simulink model "EV_thermal_charger_2015a_20200311"  (R2015a)
settings: Solver=ode3  StartTime=0.0  StopTime=1800  FixedStep=sampling_time  RelTol=1e-3
PreLoadFcn:
  | run('init_setting.m')
PostLoadFcn:
  | set_param(gcs, 'SimulationCommand', 'update');
  | load('save_param/save_P_Charger', 'P_Charger');
  | load('save_param/save_T_User_set_temp_degC','T_User_set_temp_degC');
  | load('save_param/save_ENV_PNT_PTTH_Temp_add_degC','ENV_PNT_PTTH_Temp_add_degC');
  | load('save_param/save_ENV_PNT_CABIN_Temp_add_degC','ENV_PNT_CABIN_Temp_add_degC');
  | load('save_param/save_ENV_PNT_PHI_Sunlight_W','ENV_PNT_PHI_Sunlight_W');
  | load('save_param/save_ENV_PNT_Outside_Temp_ini_degC','ENV_PNT_Outside_Temp_ini_degC');
undefined symbols (not defined in the file or in its folder): BK_PNT_Pow_UL, BK_PNT_ReGene_vel_limit_DN_kmph, BK_PNT_ReGene_vel_limit_UP_kmph, BK_PNT_Tau_brake, Brk_LL, Brk_PGain, Brk_UL, BT_PNT_Hi_C_pol_hi_batt, BT_PNT_Hi_Capa_hi_batt_F, BT_PNT_Hi_ocv_SOC_hi_batt_OCV_V_table, BT_PNT_Hi_ocv_SOC_hi_batt_OCV_V_table_x_SOC, BT_PNT_Hi_R_hi_batt_cell, BT_PNT_Hi_R_pol_hi_batt, BT_PNT_Hi_SOC_MAX_hi_batt, BT_PNT_Hi_SOC_MIN_hi_batt, BT_PNT_Hi_SOC_START_hi_batt, BT_PNT_Lo_Capa_lo_batt_F, BT_PNT_Lo_ocv_SOC_lo_batt_OCV_V_table, BT_PNT_Lo_ocv_SOC_lo_batt_OCV_V_table_x_SOC, BT_PNT_Lo_R_lo_batt_ohm, BT_PNT_Lo_SOC_MAX_lo_batt, BT_PNT_Lo_SOC_MIN_lo_batt, BT_PNT_Lo_SOC_START_lo_batt, BTTH_CNT_P_BT_Heater_W, BTTH_CNT_P_BT_Heater_W_x_BTCells_degC, BTTH_CNT_Voltage_BTFan_V, BTTH_CNT_Voltage_BTFan_V_x_BTCells_degC, BTTH_PNT_BT_Heat_Resi_KpW, BTTH_PNT_BT_Heat_Resi_KpW_x_Wind_m3ps, BTTH_PNT_BT_Heater2BTCells_Heat_Resi_KpW, BTTH_PNT_BT_Heater_Heat_Capa_JpK, BTTH_PNT_BTBlock2BTAir_Heat_Resi_KpW, BTTH_PNT_BTBlock_Heat_Capa_JpK, BTTH_PNT_BTCells2BTBlock_Heat_Resi_KpW, BTTH_PNT_BTCells_Heat_Capa_JpK, BTTH_PNT_v_BTFan_Wind_vel_mps, BTTH_PNT_v_BTFan_Wind_vel_mps_x_V_BTFan, CATH_CNT_P_Aircon_W_LL, CATH_CNT_P_Aircon_W_UL, CATH_CNT_P_Gain_Aircon, CATH_CNT_P_Gain_PTC_Heater, CATH_CNT_P_Gain_SeatHT, CATH_CNT_P_PTC_Heater, CATH_CNT_P_PTC_Heater_W_LL, CATH_CNT_P_PTC_Heater_W_UL, CATH_CNT_P_PTC_Heater_x_T_Outside_temp_degC, CATH_CNT_P_SeatHT_W_LL, CATH_CNT_P_SeatHT_W_UL, CATH_CNT_PGain_Temp_blowout, CATH_CNT_T_Aircon_Indoor_degC, CATH_CNT_T_Aircon_Indoor_degC_x_T_blowout_degC, CATH_CNT_T_PTC_Heater_degC_UL, CATH_CNT_T_SeatHT_Temp_degC, CATH_CNT_T_SeatHT_Temp_degC_x_T_blowout_degC, CATH_CNT_V_HVAC_Fan, CATH_CNT_V_HVAC_Fan_x_T_blowout_degC, CATH_CNT_V_RDFan_V, CATH_CNT_V_RDFan_x_P_Aircon_W, CATH_PNT_Air_Convection_Heat_Resi_KpW, CATH_PNT_Air_Convection_Heat_Resi_x_mps ... (+141)
undefined symbols (not defined in the file): ACC_D_Gain, ACC_I_Gain, ACC_P_Gain
libraries: METI_Lib_vehicle_model x52, simulink x35
(part 4 of 6)

== system EV_thermal_charger_2015a_20200311/Vehicle/VCU_CNT/PDfSOC ==
  note: 放電電力マップ
  note: 充電電力マップ
  SOC_BT_Hi_PNT_per : Inport
  PSoFin_map : Lookup_n-D  NumberOfTableDimensions=1  BreakpointsForDimension1=VCU_CNT_PSoFin_soc  BeginIndexSearchUsingPreviousIndexResult=on  Table=VCU_CNT_PSoFin_battpw  ExtrapMethod=Clip  UseLastTableValue=on  InternalRulePriority=Speed  RndMeth=Simplest  InputSameDT=on
  PSoFout_map : Lookup_n-D  NumberOfTableDimensions=1  BreakpointsForDimension1=VCU_CNT_PSoFout_soc  BeginIndexSearchUsingPreviousIndexResult=on  Table=VCU_CNT_PSoFout_battpw  ExtrapMethod=Clip  UseLastTableValue=on  InternalRulePriority=Speed  RndMeth=Simplest  InputSameDT=on
  PSoFin : Outport
  PSoFout : Outport  Port=2
  wires:
  PSoFout_map/1 -> PSoFout/1
  PSoFin_map/1 -> PSoFin/1
  SOC_BT_Hi_PNT_per/1 -> PSoFout_map/1, PSoFin_map/1

== system EV_thermal_charger_2015a_20200311/Vehicle/VCU_CNT/ReGenerativeBrake_Calc ==
  note: 回生ブレーキ
      | 推進力[N]
  note: 回生ブレーキ
      | モータートルク[N]
  v_VL_PNT_mps_1 : Inport
  open_break_Driver_per : Inport  Port=2
  Constant : Constant  Value=0
  Constant2 : Constant  Value=1/TM_PNT_ratio_MG2_gear
  Constant4 : Constant  Value=tire_r
  Constant5 : Constant  Value=BK_PNT_Pow_UL
  Constant9 : Constant  Value=1/DF_PNT_DF_gear
  Gain : Gain  Gain=-1
  Product1 : Product  Inputs=6
  Product2 : Product
  ReBrake_Limit_Lowspeed : Subsystem
  Saturation Dynamic : simulink/Discontinuities/Saturation Dynamic  OutMin=[]  OutMax=[]  OutDataTypeStr=Inherit: Same as second input  OutDataType=fixdt(1, 16)  OutScaling=2^-10  DoSatur=off
  eta_DF1 : Constant  Value=TM_PNT_eta_MG2_gear
  eta_DF2 : Constant  Value=DF_PNT_eta_DF
  per2F2 : Gain  Gain=1/100
  trq_R_brake_tgt : Outport
  wires:
  Saturation Dynamic/1 -> Product1/1
  Constant/1 -> Saturation Dynamic/1
  Gain/1 -> Saturation Dynamic/2
  per2F2/1 -> Product2/1
  Constant5/1 -> Product2/2
  Product2/1 -> Gain/1
  open_break_Driver_per/1 -> per2F2/1
  Constant4/1 -> Product1/2
  Constant9/1 -> Product1/3
  eta_DF2/1 -> Product1/4
  Product1/1 -> trq_R_brake_tgt/1
  Constant2/1 -> Product1/5
  eta_DF1/1 -> Product1/6
  v_VL_PNT_mps_1/1 -> ReBrake_Limit_Lowspeed/1(Vehicle_Speed_mps)
  ReBrake_Limit_Lowspeed/1(F_Brake_limit_lowspeed) -> Saturation Dynamic/3

== system EV_thermal_charger_2015a_20200311/Vehicle/VCU_CNT/trq_MG2_GuardCalc ==
  note: 回生側のトルク制限
  note: 加速側のトルク制限
  w_MG_PNT_radps : Inport
  PSoFin : Inport  Port=2
  PSoFout : Inport  Port=3
  P_HVAC_PNT_W : Inport  Port=4
  P_DCDC_PNT_W : Inport  Port=5
  Abs : Abs
  Divide_0wari : METI_Lib_vehicle_model/Divide_0wari
  Divide_0wari1 : METI_Lib_vehicle_model/Divide_0wari
  MinMax : MinMax  Function=max  Inputs=2
  MinMax1 : MinMax  Inputs=2
  MinMax2 : MinMax  Inputs=2
  MinMax3 : MinMax  Function=max  Inputs=2
  Subtract1 : Sum  Inputs=+--
  Subtract2 : Sum  Inputs=+--
  力行側出力上限 : Constant  Value=MG_CNT_Pmax_MG_Gene_W
  力行側定トルク回転数上限 : Constant  Value=MG_CNT_MG_Const_trq_Gene_radps
  回生側出力上限 : Constant  Value=MG_CNT_Pmin_MG_ReGene_W
  回生側定トルク回転数上限 : Constant  Value=MG_CNT_MG_Const_trq_ReGene_radps
  trq_MG2_UpperGuard : Outport
  trq_MG2_LowerGuard : Outport  Port=2
  wires:
  MinMax2/1 -> Divide_0wari1/1  "使用可能電力"
  w_MG_PNT_radps/1 -> Abs/1
  Divide_0wari1/1 -> trq_MG2_UpperGuard/1  "トルク上限"
  MinMax/1 -> Divide_0wari1/2, Divide_0wari/2
  Abs/1 -> MinMax/1
  MinMax1/1 -> MinMax/2
  PSoFout/1 -> Subtract1/1  "バッテリ放電電力上限値"
  P_HVAC_PNT_W/1 -> Subtract2/2, Subtract1/2
  MinMax3/1 -> Divide_0wari/1
  Divide_0wari/1 -> trq_MG2_LowerGuard/1
  PSoFin/1 -> Subtract2/1
  力行側定トルク回転数上限/1 -> MinMax1/1
  回生側定トルク回転数上限/1 -> MinMax1/2
  Subtract1/1 -> MinMax2/1  "使用可能電力"
  Subtract2/1 -> MinMax3/2
  力行側出力上限/1 -> MinMax2/2
  回生側出力上限/1 -> MinMax3/1
  P_DCDC_PNT_W/1 -> Subtract2/3, Subtract1/3

== system EV_thermal_charger_2015a_20200311/Vehicle/VCU_CNT/trq_MG2_tgtCalc2 ==
  note: ～回生協調ブレーキ時～
      | アクセルオフによる回生ブレーキトルクと
      | ブレーキ操作による回生ブレーキトルクを合算し
      | モーター要求トルクとする
  note: ～回生協調ブレーキ時～
      | モーター要求トルクから
      | アクセルオフによる回生ブレーキトルクを減算し
      | 実際に出力できているブレーキ操作による回生ブレーキトルクを算出
      | それを車両駆動力としてブレーキECUへ送信する
  User_Power_req : Inport
  w_MG_PNT_radps : Inport  Port=2
  trq_motor_UserAcc_tgt : Inport  Port=3
  trq_MG2_UpperGuard : Inport  Port=4
  trq_MG2_LowerGuard : Inport  Port=5
  trq_R_brake_tgt : Inport  Port=6
  Add : Sum
  Add1 : Sum  Inputs=+-
  Constant1 : Constant  Value=TM_PNT_ratio_MG2_gear
  Constant2 : Constant  Value=DF_PNT_DF_gear
  Constant4 : Constant  Value=1/tire_r
  Product1 : Product  Inputs=6
  Saturation Dynamic2 : simulink/Discontinuities/Saturation Dynamic  OutMin=[]  OutMax=[]  OutDataTypeStr=Inherit: Same as second input  OutDataType=fixdt(1, 16)  OutScaling=2^-10  DoSatur=off
  Saturation Dynamic4 : simulink/Discontinuities/Saturation Dynamic  OutMin=[]  OutMax=[]  OutDataTypeStr=Inherit: Same as second input  OutDataType=fixdt(1, 16)  OutScaling=2^-10  DoSatur=off
  Switch4 : Switch  Criteria=u2 > Threshold
  eta_DF1 : Constant  Value=1/DF_PNT_eta_DF
  eta_DF2 : Constant  Value=1/TM_PNT_eta_MG2_gear
  回転数上限超過時トルク制限処理 : Subsystem
  tgt_Trq_VCU_CNT_MG_Nm : Outport
  F_VCU_CNT_re_break_N : Outport  Port=2
  wires:
  Saturation Dynamic4/1 -> Add1/1, tgt_Trq_VCU_CNT_MG_Nm/1
  trq_MG2_LowerGuard/1 -> Saturation Dynamic2/3, Saturation Dynamic4/3
  回転数上限超過時トルク制限処理/1(flag_overrev) -> Switch4/2
  Add/1 -> Saturation Dynamic4/2
  trq_motor_UserAcc_tgt/1 -> 回転数上限超過時トルク制限処理/1(trq_MG2_tgt), Switch4/1
  trq_MG2_UpperGuard/1 -> Saturation Dynamic2/1, Saturation Dynamic4/1
  w_MG_PNT_radps/1 -> 回転数上限超過時トルク制限処理/2(w_ROT_motor)
  User_Power_req/1 -> 回転数上限超過時トルク制限処理/3(User_Power_req)
  回転数上限超過時トルク制限処理/2(trq_MG2_guarded) -> Switch4/3
  Add1/1 -> Product1/1
  Constant4/1 -> Product1/2
  Constant2/1 -> Product1/3
  eta_DF1/1 -> Product1/4
  Product1/1 -> F_VCU_CNT_re_break_N/1
  Switch4/1 -> Add/2, Saturation Dynamic2/2
  trq_R_brake_tgt/1 -> Add/1
  Saturation Dynamic2/1 -> Add1/2
  Constant1/1 -> Product1/5
  eta_DF2/1 -> Product1/6

== system EV_thermal_charger_2015a_20200311/Vehicle/VCU_CNT/ユーザ要求駆力算出 ==
  note: 低速時に目標出力が0にならないよう
      | 5km/h以下では車速を5km/hとして
      | 目標出力を計算するための
      | 速度切替処理
  note: モーター軸の要求トルク
  open_accel_Driver_per : Inport
  open_break_Driver_per : Inport  Port=2
  v_VL_PNT_mps_1 : Inport  Port=3
  Compare To Constant : simulink/Logic and Bit Operations/Compare To Constant  relop=<  const=VCU_CNT_trq_req_v_vehicle_th  OutDataTypeStr=boolean
  Compare To Constant1 : simulink/Logic and Bit Operations/Compare To Constant  relop=>  const=VCU_CNT_trq_req_brak_th  OutDataTypeStr=boolean
  Constant : Constant  Value=5
  Constant1 : Constant  Value=DF_PNT_DF_gear
  Constant2 : Constant  Value=TM_PNT_ratio_MG2_gear
  Constant3 : Constant  Value=VCU_CNT_trq_req_Gain_ON
  Constant4 : Constant  Value=1/tire_r
  Constant5 : Constant  Value=VCU_CNT_trq_req_Gain_OFF
  Gain1 : Gain  Gain=mps2kmph
  Logical Operator : Logic  AllPortsSameDT=off  OutDataTypeStr=boolean
  Product : Product
  Product1 : Product  Inputs=6
  Product3 : Product
  Relational Operator : RelationalOperator  Operator=>  OutDataTypeStr=boolean
  Switch : Switch  Criteria=u2 > Threshold  Threshold=0.5
  Switch1 : Switch  Criteria=u2 > Threshold  Threshold=0.5
  Transfer Fcn : TransferFcn  Denominator=[VCU_CNT_trq_req_delaytime 1]
  eta_DF1 : Constant  Value=DF_PNT_eta_DF
  eta_DF2 : Constant  Value=TM_PNT_eta_MG2_gear
  kmph2mps1 : Gain  Gain=kmph2mps
  mps2kmph : Gain  Gain=mps2kmph
  要求駆動トルク推定 : Lookup_n-D  BreakpointsForDimension1=VCU_CNT_trq_require_v_kmph  BreakpointsForDimension2=VCU_CNT_trq_require_accper  BeginIndexSearchUsingPreviousIndexResult=on  Table=VCU_CNT_trq_require_Nm  ExtrapMethod=Clip  InternalRulePriority=Speed  RndMeth=Simplest  InputSameDT=on
  P_vehicle_tgt : Outport
  trq_motor_UserAcc_tgt : Outport  Port=2
  wires:
  Switch/1 -> Product3/1
  Product3/1 -> P_vehicle_tgt/1
  Constant/1 -> kmph2mps1/1, Relational Operator/2
  mps2kmph/1 -> Relational Operator/1
  Relational Operator/1 -> Switch/2
  kmph2mps1/1 -> Switch/3
  Constant4/1 -> Product1/1
  Constant1/1 -> Product1/2
  eta_DF1/1 -> Product1/3
  Product1/1 -> Product3/2
  要求駆動トルク推定/1 -> Product1/6, Product/1
  Constant5/1 -> Switch1/1
  v_VL_PNT_mps_1/1 -> mps2kmph/1, Gain1/1, Switch/1
  open_break_Driver_per/1 -> Compare To Constant1/1
  Compare To Constant/1 -> Logical Operator/1
  Compare To Constant1/1 -> Logical Operator/2
  Logical Operator/1 -> Switch1/2
  Constant3/1 -> Switch1/3
  Switch1/1 -> Transfer Fcn/1
  Transfer Fcn/1 -> Product/2
  Product/1 -> trq_motor_UserAcc_tgt/1
  Gain1/1 -> 要求駆動トルク推定/1, Compare To Constant/1
  open_accel_Driver_per/1 -> 要求駆動トルク推定/2
  Constant2/1 -> Product1/4
  eta_DF2/1 -> Product1/5

== system EV_thermal_charger_2015a_20200311/Vehicle/VL_PNT/cal_Hill_Climbing_Resi ==
  note: 登坂抵抗
  In1 : Inport
  Constant2 : Constant  Value=g
  Constant3 : Constant  Value=M
  Gain : Gain  Gain=deg2rad
  Product1 : Product
  Product3 : Product
  Trigonometric Function : Trigonometry
  Out1 : Outport
  wires:
  Trigonometric Function/1 -> Product1/2
  Product1/1 -> Out1/1
  Product3/1 -> Product1/1
  Gain/1 -> Trigonometric Function/1
  Constant2/1 -> Product3/2
  Constant3/1 -> Product3/1
  In1/1 -> Gain/1

== system EV_thermal_charger_2015a_20200311/Driver/Caliculate_Opeining_Accel/FB/Filter ==
  In1 : Inport
  Gain3 : Gain  Gain=10
  Gain4 : Gain  Gain=0.1
  Rounding Function : Rounding  Operator=round
  Out1 : Outport
  wires:
  Rounding Function/1 -> Gain4/1
  In1/1 -> Gain3/1
  Gain3/1 -> Rounding Function/1
  Gain4/1 -> Out1/1

== system EV_thermal_charger_2015a_20200311/Driver/Caliculate_Opeining_Accel/FF1/Subsystem ==
  Req_Force : Inport
  Upper_Acc_Force_Input : Inport  Port=2
  Upper_ACC_percent : Inport  Port=3
  Lower_Acc_Force_Input : Inport  Port=4
  Lower_Acc_percent : Inport  Port=5
  Add10 : Sum
  Add11 : Sum  Inputs=+-
  Add8 : Sum  Inputs=+-
  Add9 : Sum  Inputs=+-
  Compare To Zero1 : simulink/Logic and Bit Operations/Compare To Zero  relop=>  OutDataTypeStr=boolean
  Divide_0wari2 : METI_Lib_vehicle_model/Divide_0wari
  Product2 : Product
  Acc_percent_Out : Outport
  threshold_Out : Outport  Port=2
  wires:
  Compare To Zero1/1 -> threshold_Out/1
  Req_Force/1 -> Add9/1
  Lower_Acc_Force_Input/1 -> Add9/2, Add8/2
  Add11/1 -> Product2/2
  Lower_Acc_percent/1 -> Add10/2, Add11/2
  Upper_Acc_Force_Input/1 -> Add8/1
  Product2/1 -> Add10/1
  Add8/1 -> Divide_0wari2/2
  Divide_0wari2/1 -> Product2/1
  Add9/1 -> Compare To Zero1/1, Divide_0wari2/1
  Upper_ACC_percent/1 -> Add11/1
  Add10/1 -> Acc_percent_Out/1

== system EV_thermal_charger_2015a_20200311/Driver/Caliculate_Opeining_Accel/FF1/Subsystem1 ==
  Req_Force : Inport
  Upper_Acc_Force_Input : Inport  Port=2
  Upper_ACC_percent : Inport  Port=3
  Lower_Acc_Force_Input : Inport  Port=4
  Lower_Acc_percent : Inport  Port=5
  Add10 : Sum
  Add11 : Sum  Inputs=+-
  Add8 : Sum  Inputs=+-
  Add9 : Sum  Inputs=+-
  Compare To Zero1 : simulink/Logic and Bit Operations/Compare To Zero  relop=>  OutDataTypeStr=boolean
  Divide_0wari2 : METI_Lib_vehicle_model/Divide_0wari
  Product2 : Product
  Acc_percent_Out : Outport
  threshold_Out : Outport  Port=2
  wires:
  Compare To Zero1/1 -> threshold_Out/1
  Req_Force/1 -> Add9/1
  Lower_Acc_Force_Input/1 -> Add9/2, Add8/2
  Add11/1 -> Product2/2
  Lower_Acc_percent/1 -> Add10/2, Add11/2
  Upper_Acc_Force_Input/1 -> Add8/1
  Product2/1 -> Add10/1
  Add8/1 -> Divide_0wari2/2
  Divide_0wari2/1 -> Product2/1
  Add9/1 -> Compare To Zero1/1, Divide_0wari2/1
  Upper_ACC_percent/1 -> Add11/1
  Add10/1 -> Acc_percent_Out/1

== system EV_thermal_charger_2015a_20200311/Driver/Caliculate_Opeining_Accel/FF1/Subsystem2 ==
  Req_Force : Inport
  Upper_Acc_Force_Input : Inport  Port=2
  Upper_ACC_percent : Inport  Port=3
  Lower_Acc_Force_Input : Inport  Port=4
  Lower_Acc_percent : Inport  Port=5
  Add10 : Sum
  Add11 : Sum  Inputs=+-
  Add8 : Sum  Inputs=+-
  Add9 : Sum  Inputs=+-
  Compare To Zero1 : simulink/Logic and Bit Operations/Compare To Zero  relop=>  OutDataTypeStr=boolean
  Divide_0wari2 : METI_Lib_vehicle_model/Divide_0wari
  Product2 : Product
  Acc_percent_Out : Outport
  threshold_Out : Outport  Port=2
  wires:
  Compare To Zero1/1 -> threshold_Out/1
  Req_Force/1 -> Add9/1
  Lower_Acc_Force_Input/1 -> Add9/2, Add8/2
  Add11/1 -> Product2/2
  Lower_Acc_percent/1 -> Add10/2, Add11/2
  Upper_Acc_Force_Input/1 -> Add8/1
  Product2/1 -> Add10/1
  Add8/1 -> Divide_0wari2/2
  Divide_0wari2/1 -> Product2/1
  Add9/1 -> Compare To Zero1/1, Divide_0wari2/1
  Upper_ACC_percent/1 -> Add11/1
  Add10/1 -> Acc_percent_Out/1

== system EV_thermal_charger_2015a_20200311/Driver/Caliculate_Opeining_Accel/FF1/慣性 ==
  v_tgt : Inport
  Add : Sum
  Constant : Constant  Value=M
  Constant1 : Constant  Value=1/2
  Derivative : Derivative
  Derivative1 : Derivative
  Divide1 : Product  Inputs=***
  Memory : Memory
  F_Inertia : Outport
  wires:
  Divide1/1 -> F_Inertia/1
  v_tgt/1 -> Derivative/1, Memory/1
  Add/1 -> Divide1/2
  Derivative/1 -> Add/1
  Derivative1/1 -> Add/2
  Memory/1 -> Derivative1/1
  Constant1/1 -> Divide1/1
  Constant/1 -> Divide1/3

== system EV_thermal_charger_2015a_20200311/Driver/Caliculate_Opeining_Accel/FF1/空気抵抗 ==
  v_tgt : Inport
  V_wind : Constant  Value=0
  cal_Air_resi1 : METI_Lib_vehicle_model/vehicle_model/cal_Air_resi  Vel_max=200
  F_air_resi : Outport
  wires:
  cal_Air_resi1/1 -> F_air_resi/1
  V_wind/1 -> cal_Air_resi1/2
  v_tgt/1 -> cal_Air_resi1/1

== system EV_thermal_charger_2015a_20200311/Driver/Caliculate_Opeining_Accel/FF1/転がり抵抗 ==
  v_tgt : Inport
  cal_roll_resi : METI_Lib_vehicle_model/vehicle_model/cal_roll_resi  Myu_tire=myu  Vehicle_Mass=M  Gravi_acc=g
  F_rollresi : Outport
  wires:
  cal_roll_resi/1 -> F_rollresi/1
  v_tgt/1 -> cal_roll_resi/1

== system EV_thermal_charger_2015a_20200311/Vehicle/BTTH_PNT/BB_PNT/BTBlock_Heat_Capacity ==
  ini_T_Environment_Outside_degC : Inport
  PHI_BTBlock1_W : Inport  Port=2
  PHI_BTBlock2_W : Inport  Port=3
  Add : Sum
  Add1 : Sum
  Constant : Constant  Value=BTTH_PNT_BTBlock_Heat_Capa_JpK
  Divide : Product  Inputs=/*
  Integrator : Integrator
  degC->K : Subsystem
  T_BTBlock1_K : Outport
  T_BTBlock2_K : Outport  Port=2
  wires:
  PHI_BTBlock2_W/1 -> Add/2
  PHI_BTBlock1_W/1 -> Add/1
  Constant/1 -> Divide/1
  Add/1 -> Divide/2
  Divide/1 -> Integrator/1
  ini_T_Environment_Outside_degC/1 -> degC->K/1(degC)
  Integrator/1 -> Add1/2
  Add1/1 -> T_BTBlock1_K/1, T_BTBlock2_K/1
  degC->K/1(K) -> Add1/1

== system EV_thermal_charger_2015a_20200311/Vehicle/BTTH_PNT/BB_PNT/BT_Block2Air_Heat_Resistance ==
  T_ATM_PNT_BB_K : Inport
  T_BTBlock_Resi2_K : Inport  Port=2
  Add : Sum  Inputs=+-
  Constant : Constant  Value=BTTH_PNT_BTBlock2BTAir_Heat_Resi_KpW
  Divide : Product  Inputs=*/
  Gain : Gain  Gain=-1
  Gain1 : Gain
  PHI_BT2AIR_Resi1_W : Outport
  PHI_BTBlock_Resi2_W : Outport  Port=2
  wires:
  Constant/1 -> Divide/2
  Add/1 -> Divide/1
  Divide/1 -> Gain/1, Gain1/1
  Gain/1 -> PHI_BTBlock_Resi2_W/1
  T_BTBlock_Resi2_K/1 -> Add/1
  T_ATM_PNT_BB_K/1 -> Add/2
  Gain1/1 -> PHI_BT2AIR_Resi1_W/1

== system EV_thermal_charger_2015a_20200311/Vehicle/BTTH_PNT/BC_PNT/BTCells_Heat_Capacity ==
  ini_T_Environment_Outside_degC : Inport
  PHI_BTCells1_W : Inport  Port=2
  PHI_BTCells2_W : Inport  Port=3
  PHI_BTCells3_W : Inport  Port=4
  PHI_BTCells4_W : Inport  Port=5
  Add : Sum  Inputs=++++
  Add1 : Sum
  Constant : Constant  Value=BTTH_PNT_BTCells_Heat_Capa_JpK
  Divide : Product  Inputs=/*
  Integrator : Integrator
  degC->K : Subsystem
  T_BTCells1_K : Outport
  T_BTCells2_K : Outport  Port=2
  T_BTCells3_K : Outport  Port=3
  T_BTCells4_K : Outport  Port=4
  wires:
  PHI_BTCells1_W/1 -> Add/1
  Constant/1 -> Divide/1
  Add/1 -> Divide/2
  Divide/1 -> Integrator/1
  ini_T_Environment_Outside_degC/1 -> degC->K/1(degC)
  Integrator/1 -> Add1/2
  Add1/1 -> T_BTCells4_K/1, T_BTCells3_K/1, T_BTCells1_K/1, T_BTCells2_K/1
  degC->K/1(K) -> Add1/1
  PHI_BTCells2_W/1 -> Add/2
  PHI_BTCells3_W/1 -> Add/3
  PHI_BTCells4_W/1 -> Add/4

== system EV_thermal_charger_2015a_20200311/Vehicle/BTTH_PNT/BC_PNT/BT_Cells2BTBlock_Heat_Resistance ==
  T_BTBlock_Resi1_K : Inport
  T_BTCells_Resi2_K : Inport  Port=2
  Add : Sum  Inputs=+-
  Constant : Constant  Value=BTTH_PNT_BTCells2BTBlock_Heat_Resi_KpW
  Divide : Product  Inputs=*/
  Gain : Gain  Gain=-1
  Gain1 : Gain
  PHI_BTBlock_Resi1_W : Outport
  PHI_BTCells_Resi2_W : Outport  Port=2
  wires:
  Constant/1 -> Divide/2
  Add/1 -> Divide/1
  Divide/1 -> Gain/1, Gain1/1
  T_BTCells_Resi2_K/1 -> Add/1
  T_BTBlock_Resi1_K/1 -> Add/2
  Gain1/1 -> PHI_BTBlock_Resi1_W/1
  Gain/1 -> PHI_BTCells_Resi2_W/1

== system EV_thermal_charger_2015a_20200311/Vehicle/BTTH_PNT/BF_PNT/BTFan_Heat_Resistance ==
  "BTTH_PNT_BTFan_Heat_Resi_KpW " : Inport
  T_ATM_PNT_BF_K : Inport  Port=2
  T_BT_Fan_Resi2_K : Inport  Port=3
  Add : Sum  Inputs=+-
  Divide : Product  Inputs=*/
  Gain : Gain  Gain=-1
  Gain1 : Gain
  PHI_BT_Fan_Resi1_W : Outport
  PHI_BT_Fan_Resi2_W : Outport  Port=2
  wires:
  "BTTH_PNT_BTFan_Heat_Resi_KpW "/1 -> Divide/2
  Add/1 -> Divide/1
  Divide/1 -> Gain/1, Gain1/1
  Gain/1 -> PHI_BT_Fan_Resi2_W/1
  T_BT_Fan_Resi2_K/1 -> Add/1
  T_ATM_PNT_BF_K/1 -> Add/2
  Gain1/1 -> PHI_BT_Fan_Resi1_W/1

== system EV_thermal_charger_2015a_20200311/Vehicle/BTTH_PNT/BF_PNT/BT_Fan_Heat_Resi_Calc ==
  note: ラジエターファンの動作で
      | 発生する風速
  BTTH_PNT_Voltage_BTFan_V : Inport
  1-D Lookup Table : Lookup_n-D  NumberOfTableDimensions=1  BreakpointsForDimension1=BTTH_PNT_BT_Heat_Resi_KpW_x_Wind_m3ps  Table=BTTH_PNT_BT_Heat_Resi_KpW  InternalRulePriority=Speed  RndMeth=Simplest  InputSameDT=on
  1-D Lookup Table1 : Lookup_n-D  NumberOfTableDimensions=1  BreakpointsForDimension1=BTTH_PNT_v_BTFan_Wind_vel_mps_x_V_BTFan  Table=BTTH_PNT_v_BTFan_Wind_vel_mps  InternalRulePriority=Speed  RndMeth=Simplest  InputSameDT=on
  "BTTH_PNT_BTFan_Heat_Resi_KpW " : Outport
  wires:
  BTTH_PNT_Voltage_BTFan_V/1 -> 1-D Lookup Table1/1
  1-D Lookup Table/1 -> "BTTH_PNT_BTFan_Heat_Resi_KpW "/1
  1-D Lookup Table1/1 -> 1-D Lookup Table/1

== system EV_thermal_charger_2015a_20200311/Vehicle/BTTH_PNT/BH_PNT/BT_Heater ==
  T_BT_Heater_K : Inport
  tgt_P_BTTH_CNT_BTHeater_W : Inport  Port=2
  V_BT_Lo_PNT_V : Inport  Port=3
  Divide_0wari : METI_Lib_vehicle_model/Divide_0wari
  Gain : Gain  Gain=-1
  Terminator : Terminator
  PHI_BT_Heater_W : Outport
  I_BT_Heater_A : Outport  Port=2
  wires:
  Divide_0wari/1 -> Gain/1
  tgt_P_BTTH_CNT_BTHeater_W/1 -> PHI_BT_Heater_W/1, Divide_0wari/1
  V_BT_Lo_PNT_V/1 -> Divide_0wari/2
  T_BT_Heater_K/1 -> Terminator/1
  Gain/1 -> I_BT_Heater_A/1

== system EV_thermal_charger_2015a_20200311/Vehicle/BTTH_PNT/BH_PNT/BT_Heater2BTCells_Heat_Resistance ==
  T_BTCells_Resi1_K : Inport
  T_BT_Heater_Resi2_K : Inport  Port=2
  Add : Sum  Inputs=+-
  Constant : Constant  Value=BTTH_PNT_BT_Heater2BTCells_Heat_Resi_KpW
  Divide : Product  Inputs=*/
  Gain : Gain  Gain=-1
  Gain1 : Gain
  PHI_BTCells_Resi1_W : Outport
  PHI_BT_Heater_Resi2_W : Outport  Port=2
  wires:
  Constant/1 -> Divide/2
  Add/1 -> Divide/1
  Divide/1 -> Gain/1, Gain1/1
  Gain/1 -> PHI_BT_Heater_Resi2_W/1
  T_BT_Heater_Resi2_K/1 -> Add/1
  T_BTCells_Resi1_K/1 -> Add/2
  Gain1/1 -> PHI_BTCells_Resi1_W/1

== system EV_thermal_charger_2015a_20200311/Vehicle/BTTH_PNT/BH_PNT/BT_Heater_Heat_Capacity ==
  PHI_BTCells_Resi1_W : Inport
  PHI_BT_Heater1_W : Inport  Port=2
  PHI_BT_Heater2_W : Inport  Port=3
  Add : Sum
  Add1 : Sum
  Constant : Constant  Value=BTTH_PNT_BT_Heater_Heat_Capa_JpK
  Divide : Product  Inputs=/*
  Integrator : Integrator
  degC->K : Subsystem
  T_BT_Heater1_K : Outport
  T_BT_Heater2_K : Outport  Port=2
  wires:
  PHI_BT_Heater2_W/1 -> Add/2
  PHI_BT_Heater1_W/1 -> Add/1
  Constant/1 -> Divide/1
  Add/1 -> Divide/2
  Divide/1 -> Integrator/1
  PHI_BTCells_Resi1_W/1 -> degC->K/1(degC)
  Integrator/1 -> Add1/2
  Add1/1 -> T_BT_Heater2_K/1, T_BT_Heater1_K/1
  degC->K/1(K) -> Add1/1

== system EV_thermal_charger_2015a_20200311/Vehicle/BT_Hi_PNT/Cal_SOC/Subsystem4 ==
  In1 : Inport
  In2 : Inport  Port=2
  To Workspace : ToWorkspace  VariableName=SOC_LoBat  SampleTime=-1
      settings: Decimation=num_tws_mabiki
  To Workspace1 : ToWorkspace  VariableName=Asec_LoBat  SampleTime=-1
      settings: Decimation=num_tws_mabiki
  wires:
  In1/1 -> To Workspace/1
  In2/1 -> To Workspace1/1

== system EV_thermal_charger_2015a_20200311/Vehicle/CATH_CNT/Calc_Temp_Blowout/FB ==
  T_diff_temp_degC : Inport
  Constant : Constant  Value=CATH_CNT_PGain_Temp_blowout
  Product : Product
  Q_FB : Outport
  wires:
  T_diff_temp_degC/1 -> Product/1
  Product/1 -> Q_FB/1
  Constant/1 -> Product/2

== system EV_thermal_charger_2015a_20200311/Vehicle/CATH_CNT/Calc_Temp_Blowout/FF1 ==
  note: [m2K/W]
  note: ユルゲスの実験式による
      | 対流の熱伝達率[W/m2K]を逆数にして
      | 熱抵抗[m2K/W]にしたもの
  note: [m2K/W]
  note: ユルゲスの実験式による
      | 対流の熱伝達率[W/m2K]を逆数にして
      | 熱抵抗[m2K/W]にしたもの
  note: 室内の風速
  T_Outside_temp_degC : Inport
  T_CABIN_AIR_temp_degC : Inport  Port=2
  v_vehicle_mps : Inport  Port=3
  Abs : Abs
  Add : Sum
  Air_Convection_Heat_Resi : Lookup_n-D  NumberOfTableDimensions=1  BreakpointsForDimension1=CATH_PNT_Air_Convection_Heat_Resi_x_mps  Table=CATH_PNT_Air_Convection_Heat_Resi_KpW  InternalRulePriority=Speed  RndMeth=Simplest  InputSameDT=on
  Air_Convection_Heat_Resi1 : Lookup_n-D  NumberOfTableDimensions=1  BreakpointsForDimension1=CATH_PNT_Air_Convection_Heat_Resi_x_mps  Table=CATH_PNT_Air_Convection_Heat_Resi_KpW  InternalRulePriority=Speed  RndMeth=Simplest  InputSameDT=on
  Constant1 : Constant  Value=CATH_PNT_CABIN_Glass_S_m2
  Constant2 : Constant  Value=CATH_PNT_CABIN_Glass_S_m2
  Constant3 : Constant
  Divide : Product  Inputs=*/
  Divide1 : Product  Inputs=*/
  Divide2 : Product  Inputs=*/
  Subtract : Sum  Inputs=-+
  Q_Heat_Transfar : Outport
  wires:
  T_Outside_temp_degC/1 -> Subtract/1
  T_CABIN_AIR_temp_degC/1 -> Subtract/2
  Divide1/1 -> Q_Heat_Transfar/1
  Air_Convection_Heat_Resi/1 -> Divide/1
  Abs/1 -> Air_Convection_Heat_Resi/1
  Constant1/1 -> Divide/2
  v_vehicle_mps/1 -> Abs/1
  Subtract/1 -> Divide1/1
  Air_Convection_Heat_Resi1/1 -> Divide2/1
  Constant3/1 -> Air_Convection_Heat_Resi1/1
  Constant2/1 -> Divide2/2
  Divide/1 -> Add/1
  Divide2/1 -> Add/2
  Add/1 -> Divide1/2

== system EV_thermal_charger_2015a_20200311/Vehicle/CATH_PNT/CABIN/CABIN_AIR ==
  note: 車室空気の
      | 熱容量
  note: ヒートポンプからの
      | 熱量
  note: PTCヒータからの
      | 熱量
  note: シートヒータからの
      | 熱量
  note: 直射日光からの
      | 熱量
  note: ガラスを通した
      | 外気からの熱量
  note: 不透明壁からの
      | 赤外線輻射による熱量
  note: 不透明壁を通した
      | 外気からの熱量
  note: 乗員からの
      | 熱量
  Temp_ini1 : Inport
  PHI_CABIN_Aircon_W : Inport  Port=2
  PHI_CABIN_PTC_W : Inport  Port=3
  PHI_CABIN_SeatHT_W : Inport  Port=4
  PHI_CABIN_Human_W : Inport  Port=5
  PHI_CABIN_Sunlight_W : Inport  Port=6
  PHI_CABIN_Glass_W : Inport  Port=7
  PHI_CABIN_Wall_W : Inport  Port=8
  PHI_CABIN_Radiation_W : Inport  Port=9
  Add : Sum  Inputs=++++++++
  Add1 : Sum
  Constant : Constant  Value=CATH_PNT_CABIN_AIR_Heat_Capa_JpK
  Divide : Product  Inputs=/*
  Integrator : Integrator  LowerSaturationLimit=0
  degC->K : Subsystem
  T_CABIN_AIR_temp_K1 : Outport
  T_CABIN_Aicon_K : Outport  Port=2
  T_CABIN_PTC_K : Outport  Port=3
  T_CABIN_SeatHT_K : Outport  Port=4
  T_CABIN_Glass_K : Outport  Port=5
  T_CABIN_Sunlight_K : Outport  Port=6
  T_CABIN_Wall_K : Outport  Port=7
  T_CABIN_Radiation_K : Outport  Port=8
  T_CABIN_Human_K : Outport  Port=9
  wires:
  Add1/1 -> T_CABIN_Aicon_K/1, T_CABIN_PTC_K/1, T_CABIN_SeatHT_K/1, T_CABIN_Human_K/1, T_CABIN_Wall_K/1, T_CABIN_Radiation_K/1, T_CABIN_Glass_K/1, T_CABIN_Sunlight_K/1, T_CABIN_AIR_temp_K1/1
  Constant/1 -> Divide/1
  Add/1 -> Divide/2
  Divide/1 -> Integrator/1
  Temp_ini1/1 -> degC->K/1(degC)
  Integrator/1 -> Add1/2
  degC->K/1(K) -> Add1/1
  PHI_CABIN_Aircon_W/1 -> Add/1
  PHI_CABIN_PTC_W/1 -> Add/2
  PHI_CABIN_SeatHT_W/1 -> Add/3
  PHI_CABIN_Human_W/1 -> Add/4
  PHI_CABIN_Wall_W/1 -> Add/5
  PHI_CABIN_Radiation_W/1 -> Add/6
  PHI_CABIN_Glass_W/1 -> Add/7
  PHI_CABIN_Sunlight_W/1 -> Add/8

== system EV_thermal_charger_2015a_20200311/Vehicle/CATH_PNT/CABIN/GLASS ==
  note: 室内の風速
  V_vehicle_mps : Inport
  Temp_ini : Inport  Port=2
  T_GLASS2AIR_K : Inport  Port=3
  PHI_GLASS_Sunlight2_W : Inport  Port=4
  T_GLASS_CABIN_K : Inport  Port=5
  T_GLASS_Sunlight1_K : Inport  Port=6
  CABIN_Glass_Heat_Capacity : Subsystem
  CABIN_Glass_Heat_Resistance : Subsystem
  CABIN_Glass_Heat_Resistance1 : Subsystem
  Constant : Constant  Value=5
  PHI_GLASS2AIR_W : Outport
  T_GLASS_Sunlight2_K : Outport  Port=2
  PHI_GLASS_Sunlight1_W : Outport  Port=3
  PHI_GLASS_CABIN_W : Outport  Port=4
  wires:
  CABIN_Glass_Heat_Resistance/1(PHI_CABIN_Glass_Resi1_W) -> PHI_GLASS2AIR_W/1
  T_GLASS2AIR_K/1 -> CABIN_Glass_Heat_Resistance/2(T_CABIN_Glass_Resi1_K)
  CABIN_Glass_Heat_Capacity/2(T_CABIN_Glass1_K) -> CABIN_Glass_Heat_Resistance1/3(T_CABIN_Glass_Resi3_K)
  CABIN_Glass_Heat_Resistance1/2(PHI_CABIN_Glass_Resi3_W) -> CABIN_Glass_Heat_Capacity/2(PHI_CABIN_Glass1_W)
  CABIN_Glass_Heat_Capacity/1(T_CABIN_Glass2_K) -> CABIN_Glass_Heat_Resistance/3(T_CABIN_Glass_Resi2_K)
  CABIN_Glass_Heat_Resistance/2(PHI_CABIN_Glass_Resi2_W) -> CABIN_Glass_Heat_Capacity/3(PHI_CABIN_Glass2_W)
  PHI_GLASS_Sunlight2_W/1 -> PHI_GLASS_Sunlight1_W/1
  T_GLASS_Sunlight1_K/1 -> T_GLASS_Sunlight2_K/1
  Temp_ini/1 -> CABIN_Glass_Heat_Capacity/1(Temp_ini)
  T_GLASS_CABIN_K/1 -> CABIN_Glass_Heat_Resistance1/2(T_CABIN_Glass_Resi4_K)
  CABIN_Glass_Heat_Resistance1/1(PHI_CABIN_Glass_Resi4_W) -> PHI_GLASS_CABIN_W/1
  Constant/1 -> CABIN_Glass_Heat_Resistance1/1(V_wind)
  V_vehicle_mps/1 -> CABIN_Glass_Heat_Resistance/1(V_wind)

== system EV_thermal_charger_2015a_20200311/Vehicle/CATH_PNT/CABIN/Human_Thermal ==
  T_Human_Thermal_K : Inport
  Constant : Constant  Value=CATH_PNT_PHI_Human_body_W
  Terminator : Terminator
  PHI_Human_Thermal_W : Outport
  wires:
  Constant/1 -> PHI_Human_Thermal_W/1
  T_Human_Thermal_K/1 -> Terminator/1

== system EV_thermal_charger_2015a_20200311/Vehicle/CATH_PNT/CABIN/K->degC ==
  K : Inport
  Constant2 : Constant  Value=K2degC
  Sum : Sum  Inputs=++|
  degC : Outport
  wires:
  K/1 -> Sum/2
  Constant2/1 -> Sum/1
  Sum/1 -> degC/1

== system EV_thermal_charger_2015a_20200311/Vehicle/CATH_PNT/CABIN/K->degC1 ==
  K : Inport
  Constant2 : Constant  Value=K2degC
  Sum : Sum  Inputs=++|
  degC : Outport
  wires:
  K/1 -> Sum/2
  Constant2/1 -> Sum/1
  Sum/1 -> degC/1

== system EV_thermal_charger_2015a_20200311/Vehicle/CATH_PNT/CABIN/K->degC2 ==
  K : Inport
  Constant2 : Constant  Value=K2degC
  Sum : Sum  Inputs=++|
  degC : Outport
  wires:
  K/1 -> Sum/2
  Constant2/1 -> Sum/1
  Sum/1 -> degC/1

== system EV_thermal_charger_2015a_20200311/Vehicle/CATH_PNT/CABIN/K->degC3 ==
  K : Inport
  Constant2 : Constant  Value=K2degC
  Sum : Sum  Inputs=++|
  degC : Outport
  wires:
  K/1 -> Sum/2
  Constant2/1 -> Sum/1
  Sum/1 -> degC/1

== system EV_thermal_charger_2015a_20200311/Vehicle/CATH_PNT/CABIN/WALL ==
  note: 室内の風速
  V_vehicle_mps : Inport
  Temp_ini : Inport  Port=2
  T_WALL2AIR_K : Inport  Port=3
  PHI_WALL_Radiation_W : Inport  Port=4
  T_WALL_CABIN_K : Inport  Port=5
  T_WALL_Radiation1_K : Inport  Port=6
  CABIN_Wall_Heat_Capacity : Subsystem
  CABIN_Wall_Heat_Resistance : Subsystem
  CABIN_Wall_Heat_Resistance1 : Subsystem
  Constant1 : Constant  Value=5
  PHI_WALL2AIR_W : Outport
  T_WALL_Radiation_K : Outport  Port=2
  PHI_WALL_CABIN_W : Outport  Port=3
  PHI_WALL_Radiation1_W : Outport  Port=4
  wires:
  CABIN_Wall_Heat_Resistance/1(PHI_Wall_Resi1_W) -> PHI_WALL2AIR_W/1
  T_WALL2AIR_K/1 -> CABIN_Wall_Heat_Resistance/2(T_Wall_Resi1_K)
  CABIN_Wall_Heat_Capacity/2(T_CABIN_Wall1_K) -> CABIN_Wall_Heat_Resistance1/3(T_CABIN_Wall_Resi1_K)
  CABIN_Wall_Heat_Resistance1/2(PHI_CABIN_Wall_Resi1_W) -> CABIN_Wall_Heat_Capacity/2(PHI_CABIN_Wall1_W)
  CABIN_Wall_Heat_Capacity/1(T_CABIN_Wall2_K) -> CABIN_Wall_Heat_Resistance/3(T_Wall_Resi2_K)
  CABIN_Wall_Heat_Resistance/2(PHI_Wall_Resi2_W) -> CABIN_Wall_Heat_Capacity/3(PHI_CABIN_Wall2_W)
  Temp_ini/1 -> CABIN_Wall_Heat_Capacity/1(Temp_ini)
  T_WALL_CABIN_K/1 -> CABIN_Wall_Heat_Resistance1/2(T_CABIN_Wall_Resi2_K)
  CABIN_Wall_Heat_Resistance1/1(PHI_CABIN_Wall_Resi2_W) -> PHI_WALL_CABIN_W/1
  Constant1/1 -> CABIN_Wall_Heat_Resistance1/1(V_wind)
  V_vehicle_mps/1 -> CABIN_Wall_Heat_Resistance/1(V_wind)
  T_WALL_Radiation1_K/1 -> T_WALL_Radiation_K/1
  PHI_WALL_Radiation_W/1 -> PHI_WALL_Radiation1_W/1

== system EV_thermal_charger_2015a_20200311/Vehicle/CATH_PNT/HVAC/Aircon ==
  note: 室外機の
      | 熱容量
  note: 室内機の
      | 熱容量
  P_Heatpomp_Power : Inport
  Temp_ini : Inport  Port=2
  V_Aircon_V : Inport  Port=3
  PHI_Aircon_Outdoor1_W : Inport  Port=4
  PHI_Aircon_Indoor1_W : Inport  Port=5
  Aircon_Indoor_Unit_Heat_Capacity1 : Subsystem
  Aircon_Outdoor_Unit_Heat_Capacity : Subsystem
  Gain1 : Gain  Gain=-1
  K->degC : Subsystem
  K->degC1 : Subsystem
  Product1 : Product
  Switching_Air_Conditioning_Circuit : Subsystem
  T_Aircon_Outdoor_degC : Outport
  T_Aircon_Indoor_degC : Outport  Port=2
  T_Aircon_Outdoor1_K : Outport  Port=3
  T_Aircon_Indoor1_K : Outport  Port=4
  I_Aircon_A : Outport  Port=5
  tag scope: tScope_PHI_Aircon_Indoor1=global, tScope_PHI_Aircon_Outdoor1=global, tScope_P_Aircon=global
  wires:
  Aircon_Indoor_Unit_Heat_Capacity1/1(T_Aircon_Indoor2_K) -> T_Aircon_Indoor1_K/1, K->degC1/1(K)
  PHI_Aircon_Indoor1_W/1 -> [tScope_PHI_Aircon_Indoor1], Aircon_Indoor_Unit_Heat_Capacity1/3(PHI_Aircon_Indoor2_W)
  Aircon_Outdoor_Unit_Heat_Capacity/1(T_Aircon_Outdoor2_K) -> T_Aircon_Outdoor1_K/1, K->degC/1(K)
  PHI_Aircon_Outdoor1_W/1 -> Aircon_Outdoor_Unit_Heat_Capacity/3(PHI_Aircon_Outdoor2_W), [tScope_PHI_Aircon_Outdoor1]
  Temp_ini/1 -> Aircon_Outdoor_Unit_Heat_Capacity/1(Temp_ini), Aircon_Indoor_Unit_Heat_Capacity1/1(Temp_ini)
  K->degC/1(degC) -> T_Aircon_Outdoor_degC/1
  K->degC1/1(degC) -> T_Aircon_Indoor_degC/1
  Aircon_Outdoor_Unit_Heat_Capacity/2(T_Aircon_Outdoor3_K) -> Switching_Air_Conditioning_Circuit/4(T_Aircon_Outdoor4_K)
  Aircon_Indoor_Unit_Heat_Capacity1/2(T_Aircon_Indoor3_K) -> Switching_Air_Conditioning_Circuit/3(T_Aircon_Indoor4_K)
  P_Heatpomp_Power/1 -> Switching_Air_Conditioning_Circuit/2(P_Heatpomp_Power)
  V_Aircon_V/1 -> Switching_Air_Conditioning_Circuit/1(V_Compressor_V), Product1/1
  Switching_Air_Conditioning_Circuit/1(I_Compressor_A) -> I_Aircon_A/1, Gain1/1
  Product1/1 -> [tScope_P_Aircon]
  Gain1/1 -> Product1/2
  Switching_Air_Conditioning_Circuit/2(PHI_Aircon_Outdoor4_W) -> Aircon_Outdoor_Unit_Heat_Capacity/2(PHI_Aircon_Outdoor3_W)
  Switching_Air_Conditioning_Circuit/3(PHI_Aircon_Indoor4_W) -> Aircon_Indoor_Unit_Heat_Capacity1/2(PHI_Aircon_Indoor3_W)

== system EV_thermal_charger_2015a_20200311/Vehicle/CATH_PNT/HVAC/Aircon_Fan_Heat_Resi_Calc ==
  note: ラジエターファンの動作で
      | ラジエターコアに当たる風量
  CATH_PNT_Voltage_HVAC_Fan_V : Inport
  1-D Lookup Table : Lookup_n-D  NumberOfTableDimensions=1  BreakpointsForDimension1=CATH_PNT_HVAC_Heat_Resi_KpW_x_Wind_m3ps  Table=CATH_PNT_HVAC_Heat_Resi_KpW  InternalRulePriority=Speed  RndMeth=Simplest  InputSameDT=on
  1-D Lookup Table1 : Lookup_n-D  NumberOfTableDimensions=1  BreakpointsForDimension1=CATH_PNT_v_HVAC_Fan_Wind_vel_m3ps_x_V_HVAC_Fan  Table=CATH_PNT_v_HVAC_Fan_Wind_vel_m3ps  InternalRulePriority=Speed  RndMeth=Simplest  InputSameDT=on
  "HVAC_Fan_Heat_Resi_KpW " : Outport
  wires:
  CATH_PNT_Voltage_HVAC_Fan_V/1 -> 1-D Lookup Table1/1
  1-D Lookup Table/1 -> "HVAC_Fan_Heat_Resi_KpW "/1
  1-D Lookup Table1/1 -> 1-D Lookup Table/1

== system EV_thermal_charger_2015a_20200311/Vehicle/CATH_PNT/HVAC/Aircon_Heat_Resistance ==
  "Aircon_Heat_Resi_KpW " : Inport
  T_Aircon_Resi1_K : Inport  Port=2
  T_Aircon_Resi2_K : Inport  Port=3
  Add : Sum  Inputs=+-
  Divide : Product  Inputs=*/
  Gain : Gain  Gain=-1
  Gain1 : Gain
  PHI_Aircon_Resi1_W : Outport
  PHI_Aircon_Resi2_W : Outport  Port=2
  wires:
  "Aircon_Heat_Resi_KpW "/1 -> Divide/2
  Add/1 -> Divide/1
  Divide/1 -> Gain1/1, Gain/1
  Gain/1 -> PHI_Aircon_Resi2_W/1
  T_Aircon_Resi2_K/1 -> Add/1
  T_Aircon_Resi1_K/1 -> Add/2
  Gain1/1 -> PHI_Aircon_Resi1_W/1

== system EV_thermal_charger_2015a_20200311/Vehicle/CATH_PNT/HVAC/Aircon_Heat_Resistance1 ==
  "Aircon_Heat_Resi_KpW " : Inport
  T_Aircon_Resi3_K : Inport  Port=2
  T_Aircon_Resi4_K : Inport  Port=3
  Add : Sum  Inputs=+-
  Divide : Product  Inputs=*/
  Gain : Gain  Gain=-1
  Gain1 : Gain
  PHI_Aircon_Resi3_W : Outport
  PHI_Aircon_Resi4_W : Outport  Port=2
  wires:
  "Aircon_Heat_Resi_KpW "/1 -> Divide/2
  Add/1 -> Divide/1
  Divide/1 -> Gain1/1, Gain/1
  Gain/1 -> PHI_Aircon_Resi4_W/1
  T_Aircon_Resi4_K/1 -> Add/1
  T_Aircon_Resi3_K/1 -> Add/2
  Gain1/1 -> PHI_Aircon_Resi3_W/1

== system EV_thermal_charger_2015a_20200311/Vehicle/CATH_PNT/HVAC/PTC_Heater1 ==
  note: エアコン用PTCヒーター
      | 熱容量
  P_PTC_Heater_Power : Inport
  Temp_ini : Inport  Port=2
  V_PTC_Heater1_V : Inport  Port=3
  PHI_PTC_Heater1_W : Inport  Port=4
  K->degC : Subsystem
  PTC_Heater : Subsystem
  PTC_Heater_Heat_Capacity : Subsystem
  T_PTC_Heater_degC : Outport
  T_PTC_Heater1_K : Outport  Port=2
  I_PTC_Heater1_A : Outport  Port=3
  wires:
  PTC_Heater_Heat_Capacity/2(T_PTC_Heater3_K) -> PTC_Heater/3(T_PTC_Heater4_K)
  PTC_Heater_Heat_Capacity/1(T_PTC_Heater2_K) -> T_PTC_Heater1_K/1, K->degC/1(K)
  PHI_PTC_Heater1_W/1 -> PTC_Heater_Heat_Capacity/3(PHI_PTC_Heater2_W)
  Temp_ini/1 -> PTC_Heater_Heat_Capacity/1(Temp_ini)
  K->degC/1(degC) -> T_PTC_Heater_degC/1
  P_PTC_Heater_Power/1 -> PTC_Heater/1(P_PTC_Heater_Power)
  V_PTC_Heater1_V/1 -> PTC_Heater/2(V_PTC_Heater4_V)
  PTC_Heater/2(I_PTC_Heater4_A) -> I_PTC_Heater1_A/1
  PTC_Heater/1(PHI_PTC_Heater4_W) -> PTC_Heater_Heat_Capacity/2(PHI_PTC_Heater3_W)

== system EV_thermal_charger_2015a_20200311/Vehicle/CATH_PNT/HVAC/RDCoolant2Air_Heat_Resistance1 ==
  "Aircon_Air_Heat_Resi_KpW " : Inport
  T_Aircon_Air_Resi1_K : Inport  Port=2
  T_Aircon_Air_Resi2_K : Inport  Port=3
  Add : Sum  Inputs=+-
  Divide : Product  Inputs=*/
  Gain : Gain  Gain=-1
  Gain1 : Gain
  PHI_Aircon_Air_Resi1_W : Outport
  PHI_Aircon_Air_Resi2_W : Outport  Port=2
  wires:
  "Aircon_Air_Heat_Resi_KpW "/1 -> Divide/2
  Add/1 -> Divide/1
  Divide/1 -> Gain1/1, Gain/1
  Gain/1 -> PHI_Aircon_Air_Resi2_W/1
  T_Aircon_Air_Resi2_K/1 -> Add/1
  T_Aircon_Air_Resi1_K/1 -> Add/2
  Gain1/1 -> PHI_Aircon_Air_Resi1_W/1

== system EV_thermal_charger_2015a_20200311/Vehicle/CATH_PNT/Seat_Heater/K->degC ==
  K : Inport
  Constant2 : Constant  Value=K2degC
  Sum : Sum  Inputs=++|
  degC : Outport
  wires:
  K/1 -> Sum/2
  Constant2/1 -> Sum/1
  Sum/1 -> degC/1

== system EV_thermal_charger_2015a_20200311/Vehicle/CATH_PNT/Seat_Heater/SeatHT_Heat_Capacity ==
  Temp_ini : Inport
  PHI_SeatHT1_W : Inport  Port=2
  PHI_SeatHT2_W : Inport  Port=3
  Add : Sum
  Add1 : Sum
  Constant : Constant  Value=CATH_PNT_Seat_Heater_Capa_JpK
  Divide : Product  Inputs=/*
  Integrator : Integrator
  degC->K : Subsystem
  T_SeatHT2_K : Outport
  T_SeatHT1_K : Outport  Port=2
  wires:
  PHI_SeatHT2_W/1 -> Add/2
  PHI_SeatHT1_W/1 -> Add/1
  Constant/1 -> Divide/1
  Add/1 -> Divide/2
  Divide/1 -> Integrator/1
  Temp_ini/1 -> degC->K/1(degC)
  Integrator/1 -> Add1/2
  Add1/1 -> T_SeatHT1_K/1, T_SeatHT2_K/1
  degC->K/1(K) -> Add1/1

== system EV_thermal_charger_2015a_20200311/Vehicle/CATH_PNT/Seat_Heater/Seat_HT ==
  P_Seat_Heater_Power : Inport
  V_Seat_HT_V : Inport  Port=2
  T_Seat_HT_K : Inport  Port=3
  Divide_0wari : METI_Lib_vehicle_model/Divide_0wari
  Gain : Gain  Gain=-1
  Terminator : Terminator
  PHI_Seat_HT_W : Outport
  I_Seat_HT_A : Outport  Port=2
  wires:
  P_Seat_Heater_Power/1 -> PHI_Seat_HT_W/1, Divide_0wari/1
  V_Seat_HT_V/1 -> Divide_0wari/2
  Divide_0wari/1 -> Gain/1
  Gain/1 -> I_Seat_HT_A/1
  T_Seat_HT_K/1 -> Terminator/1

== system EV_thermal_charger_2015a_20200311/Vehicle/CATH_PNT/Seat_Heater/Seat_Heater_Heat_Resistance ==
  T_SeatHT_Resi2_K : Inport
  T_SeatHT_Resi1_K : Inport  Port=2
  Add : Sum  Inputs=+-
  Constant : Constant  Value=CATH_PNT_CABIN_SeatHT_Heat_Resi_KpW
  Divide : Product  Inputs=*/
  Gain : Gain  Gain=-1
  Gain1 : Gain
  PHI_SeatHT_Resi1_W : Outport
  PHI_SeatHT_Resi2_W : Outport  Port=2
  wires:
  Constant/1 -> Divide/2
  Add/1 -> Divide/1
  Divide/1 -> Gain1/1, Gain/1
  Gain/1 -> PHI_SeatHT_Resi2_W/1
  T_SeatHT_Resi2_K/1 -> Add/1
  T_SeatHT_Resi1_K/1 -> Add/2
  Gain1/1 -> PHI_SeatHT_Resi1_W/1

== system EV_thermal_charger_2015a_20200311/Vehicle/CHG_CNT/Charge_Current_calc/Initial_Charge ==
  In1 : Inport
  Action Port : ActionPort  ActionType=elseif
  Out1 : Outport
  wires:
  In1/1 -> Out1/1

== system EV_thermal_charger_2015a_20200311/Vehicle/CHG_CNT/Charge_Current_calc/Negotiation_time ==
  Action Port : ActionPort  ActionType=then
  Constant : Constant  Value=0
  Out1 : Outport
  wires:
  Constant/1 -> Out1/1

== system EV_thermal_charger_2015a_20200311/Vehicle/CHG_CNT/Charge_Current_calc/Normal_Charge ==
  note: 一定電流充電モード（CC)
      | 一定電力充電モード（CP)
      | 一定電圧充電モード（CV)
      | の三者で目標電流値を算出し、
      | その中で最も小さい電流値だったものを採用する。
  Maximum_Charge_Current_A : Inport
  Maximum_Charge_Power_W : Inport  Port=2
  Maximum_Charge_Voltage_V : Inport  Port=3
  Battery_Voltage_V : Inport  Port=4
  SOC_HiBatt : Inport  Port=5
  Maximum_Hi_Batt_SOC : Inport  Port=6
  Action Port : ActionPort  ActionType=else
  Constant_Current_Charge : Subsystem
  Constant_Power_Charge : Subsystem
  Constant_Voltage_Charge : Subsystem
  Memory : Memory
  MinMax : MinMax  Inputs=3
  Relational Operator : RelationalOperator  Operator===  OutDataTypeStr=boolean
  Current_tgt : Outport
  wires:
  Maximum_Charge_Current_A/1 -> Constant_Current_Charge/1(Maximum_Charge_Current_A), Constant_Voltage_Charge/1(Maximum_Charge_Current_A)
  MinMax/1 -> Relational Operator/1, Current_tgt/1
  Maximum_Charge_Power_W/1 -> Constant_Power_Charge/1(Maximum_Charge_Power_W)
  Constant_Current_Charge/1(Current_tgt) -> MinMax/1
  Battery_Voltage_V/1 -> Constant_Power_Charge/2(Battery_Voltage_V), Constant_Voltage_Charge/4(Battery_Voltage_V)
  Constant_Power_Charge/1(Current_tgt) -> MinMax/2
  Constant_Voltage_Charge/1(Current_tgt) -> Relational Operator/2, MinMax/3
  Memory/1 -> Constant_Voltage_Charge/5(old_mode)
  Relational Operator/1 -> Memory/1
  Maximum_Hi_Batt_SOC/1 -> Constant_Voltage_Charge/3(Maximum_Hi_Batt_SOC)
  Maximum_Charge_Voltage_V/1 -> Constant_Voltage_Charge/2(Maximum_Charge_Voltage_V)
  SOC_HiBatt/1 -> Constant_Current_Charge/2(SOC_HiBatt)

== system EV_thermal_charger_2015a_20200311/Vehicle/ELTH_PNT/INVTH_PNT/INVBlock2Air_Heat_Resistance ==
  T_INV2Air_Resi1_K : Inport
  T_INVBlock_Resi3_K : Inport  Port=2
  Add : Sum  Inputs=+-
  Constant : Constant  Value=ELTH_PNT_INVBlock2DFAir_Heat_Resi_KpW
  Divide : Product  Inputs=*/
  Gain : Gain  Gain=-1
  Gain1 : Gain
  PHI_INV2Air_Resi1_W : Outport
  PHI_INVBlock_Resi3_W : Outport  Port=2
  wires:
  Constant/1 -> Divide/2
  Add/1 -> Divide/1
  Divide/1 -> Gain1/1, Gain/1
  Gain/1 -> PHI_INVBlock_Resi3_W/1
  T_INVBlock_Resi3_K/1 -> Add/1
  T_INV2Air_Resi1_K/1 -> Add/2
  Gain1/1 -> PHI_INV2Air_Resi1_W/1

== system EV_thermal_charger_2015a_20200311/Vehicle/ELTH_PNT/INVTH_PNT/INVBlock_Heat_Capacity ==
  PHI_INVBlock2_W : Inport
  Temp_ini : Inport  Port=2
  PHI_INVBlock1_W : Inport  Port=3
  PHI_INVBlock3_W : Inport  Port=4
  Add : Sum  Inputs=+++
  Add1 : Sum
  Constant : Constant  Value=ELTH_PNT_INVBlock_Heat_Capa_JpK
  Divide : Product  Inputs=/*
  Integrator : Integrator
  degC->K : Subsystem
  T_INVBlock2_K : Outport
  T_INVBlock3_K : Outport  Port=2
  T_INVBlock1_K : Outport  Port=3
  wires:
  PHI_INVBlock1_W/1 -> Add/1
  Constant/1 -> Divide/1
  Add/1 -> Divide/2
  Divide/1 -> Integrator/1
  Temp_ini/1 -> degC->K/1(degC)
  Integrator/1 -> Add1/2
  Add1/1 -> T_INVBlock3_K/1, T_INVBlock2_K/1, T_INVBlock1_K/1
  PHI_INVBlock2_W/1 -> Add/2
  PHI_INVBlock3_W/1 -> Add/3
  degC->K/1(K) -> Add1/1

== system EV_thermal_charger_2015a_20200311/Vehicle/ELTH_PNT/INVTH_PNT/INVHeatsink2INVBlock_Heat_Resistance ==
  T_INVHeatsink_Resi2_K : Inport
  T_INVBlock_Resi1_K : Inport  Port=2
  Add : Sum  Inputs=+-
  Constant : Constant  Value=ELTH_PNT_INVHeatsink2INVBlock_Heat_Resi_KpW
  Divide : Product  Inputs=*/
  Gain : Gain  Gain=-1
  Gain1 : Gain
  PHI_INVBlock_Resi1_W : Outport
  PHI_INVHeatsink_Resi2_W : Outport  Port=2
  wires:
  Constant/1 -> Divide/2
  Add/1 -> Divide/1
  Divide/1 -> Gain1/1, Gain/1
  Gain/1 -> PHI_INVHeatsink_Resi2_W/1
  T_INVHeatsink_Resi2_K/1 -> Add/1
  T_INVBlock_Resi1_K/1 -> Add/2
  Gain1/1 -> PHI_INVBlock_Resi1_W/1

== system EV_thermal_charger_2015a_20200311/Vehicle/ELTH_PNT/INVTH_PNT/INVTH_Heatsink_Heat_Capacity ==
  Temp_ini : Inport
  PHI_INVTH_Heatsink1_W : Inport  Port=2
  PHI_INVTH_Heatsink3_W : Inport  Port=3
  PHI_INVTH_Heatsink2_W : Inport  Port=4
  Add : Sum  Inputs=+++
  Add1 : Sum
  Constant : Constant  Value=ELTH_PNT_INVHeatsink_Heat_Capa_JpK
  Divide : Product  Inputs=/*
  Integrator : Integrator
  degC->K : Subsystem
  T_INVTH_Heatsink1_K : Outport
  T_INVTH_Heatsink2_K : Outport  Port=2
  T_INVTH_Heatsink3_K : Outport  Port=3
  wires:
  PHI_INVTH_Heatsink2_W/1 -> Add/3
  PHI_INVTH_Heatsink1_W/1 -> Add/1
  Constant/1 -> Divide/1
  Add/1 -> Divide/2
  Divide/1 -> Integrator/1
  Temp_ini/1 -> degC->K/1(degC)
  Integrator/1 -> Add1/2
  Add1/1 -> T_INVTH_Heatsink3_K/1, T_INVTH_Heatsink2_K/1, T_INVTH_Heatsink1_K/1
  degC->K/1(K) -> Add1/1
  PHI_INVTH_Heatsink3_W/1 -> Add/2

== system EV_thermal_charger_2015a_20200311/Vehicle/ELTH_PNT/INVTH_PNT/K->degC1 ==
  K : Inport
  Constant2 : Constant  Value=K2degC
  Sum : Sum  Inputs=++|
  degC : Outport
  wires:
  K/1 -> Sum/2
  Constant2/1 -> Sum/1
  Sum/1 -> degC/1

== system EV_thermal_charger_2015a_20200311/Vehicle/ELTH_PNT/INVTH_PNT/K->degC2 ==
  K : Inport
  Constant2 : Constant  Value=K2degC
  Sum : Sum  Inputs=++|
  degC : Outport
  wires:
  K/1 -> Sum/2
  Constant2/1 -> Sum/1
  Sum/1 -> degC/1

== system EV_thermal_charger_2015a_20200311/Vehicle/ELTH_PNT/INVTH_PNT/MG2INVBlock_Heat_Resistance ==
  T_INVBlock_Resi2_K : Inport
  T_MGBlock_Resi4_K : Inport  Port=2
  Add : Sum  Inputs=+-
  Constant : Constant  Value=ELTH_PNT_MG2INVBlock_Heat_Resi_KpW
  Divide : Product  Inputs=*/
  Gain : Gain  Gain=-1
  Gain1 : Gain
  PHI_INVBlock_Resi2_W : Outport
  PHI_MGBlock_Resi4_W : Outport  Port=2
  wires:
  Constant/1 -> Divide/2
  Add/1 -> Divide/1
  Divide/1 -> Gain1/1, Gain/1
  Gain/1 -> PHI_MGBlock_Resi4_W/1
  T_MGBlock_Resi4_K/1 -> Add/1
  T_INVBlock_Resi2_K/1 -> Add/2
  Gain1/1 -> PHI_INVBlock_Resi2_W/1

== system EV_thermal_charger_2015a_20200311/Vehicle/ELTH_PNT/MGTH_PNT/Coil_Heat_Capacity ==
  Temp_ini : Inport
  PHI_MGCoil1_W : Inport  Port=2
  PHI_MGCoil2_W : Inport  Port=3
  Add : Sum
  Add1 : Sum
  Constant : Constant  Value=ELTH_PNT_MGCoil_Heat_Capa_JpK
  Divide : Product  Inputs=/*
  Integrator : Integrator
  degC->K : Subsystem
  T_MGCoil1_K : Outport
  T_MGCoil2_K : Outport  Port=2
  wires:
  PHI_MGCoil2_W/1 -> Add/2
  PHI_MGCoil1_W/1 -> Add/1
  Constant/1 -> Divide/1
  Add/1 -> Divide/2
  Divide/1 -> Integrator/1
  Temp_ini/1 -> degC->K/1(degC)
  Integrator/1 -> Add1/2
  Add1/1 -> T_MGCoil1_K/1, T_MGCoil2_K/1
  degC->K/1(K) -> Add1/1

== system EV_thermal_charger_2015a_20200311/Vehicle/ELTH_PNT/MGTH_PNT/K->degC1 ==
  K : Inport
  Constant2 : Constant  Value=K2degC
  Sum : Sum  Inputs=++|
  degC : Outport
  wires:
  K/1 -> Sum/2
  Constant2/1 -> Sum/1
  Sum/1 -> degC/1

== system EV_thermal_charger_2015a_20200311/Vehicle/ELTH_PNT/MGTH_PNT/K->degC2 ==
  K : Inport
  Constant2 : Constant  Value=K2degC
  Sum : Sum  Inputs=++|
  degC : Outport
  wires:
  K/1 -> Sum/2
  Constant2/1 -> Sum/1
  Sum/1 -> degC/1

== system EV_thermal_charger_2015a_20200311/Vehicle/ELTH_PNT/MGTH_PNT/MGCoil2MGHousing_Heat_Resistance ==
  T_MGCoil_Resi4_K : Inport
  T_MGHousing_Resi1_K : Inport  Port=2
  Add : Sum  Inputs=+-
  Constant : Constant  Value=ELTH_PNT_MGCoil2MGHousing_Heat_Resi_KpW
  Divide : Product  Inputs=*/
  Gain : Gain  Gain=-1
  Gain1 : Gain
  PHI_MGHousing_Resi1_W : Outport
  PHI_MGCoil_Resi4_W : Outport  Port=2
  wires:
  Constant/1 -> Divide/2
  Add/1 -> Divide/1
  Divide/1 -> Gain/1, Gain1/1
  Gain/1 -> PHI_MGCoil_Resi4_W/1
  T_MGCoil_Resi4_K/1 -> Add/1
  T_MGHousing_Resi1_K/1 -> Add/2
  Gain1/1 -> PHI_MGHousing_Resi1_W/1

== system EV_thermal_charger_2015a_20200311/Vehicle/ELTH_PNT/MGTH_PNT/MGHousing2Air_Heat_Resistance ==
  T_MG2Air_Resi1_K : Inport
  T_MGHousing_Resi5_K : Inport  Port=2
  Add : Sum  Inputs=+-
  Constant : Constant  Value=ELTH_PNT_MGHousing2TMAir_Heat_Resi_KpW
  Divide : Product  Inputs=*/
  Gain : Gain  Gain=-1
  Gain1 : Gain
  PHI_MG2Air_Resi1_W : Outport
  PHI_MGHousing_Resi5_W : Outport  Port=2
  wires:
  Constant/1 -> Divide/2
  Add/1 -> Divide/1
  Divide/1 -> Gain1/1, Gain/1
  Gain/1 -> PHI_MGHousing_Resi5_W/1
  T_MGHousing_Resi5_K/1 -> Add/1
  T_MG2Air_Resi1_K/1 -> Add/2
  Gain1/1 -> PHI_MG2Air_Resi1_W/1

== system EV_thermal_charger_2015a_20200311/Vehicle/ELTH_PNT/MGTH_PNT/MGHousing_Heat_Capacity ==
  PHI_MGHousing2_W : Inport
  PHI_MGHousing3_W : Inport  Port=2
  PHI_MGHousing4_W : Inport  Port=3
  Temp_ini : Inport  Port=4
  PHI_MGHousing1_W : Inport  Port=5
  PHI_MGHousing5_W : Inport  Port=6
  Add : Sum  Inputs=+++++
  Add1 : Sum
  Constant : Constant  Value=ELTH_PNT_MGHousing_Heat_Capa_JpK
  Divide : Product  Inputs=/*
  Integrator : Integrator
  degC->K : Subsystem
  T_MGHousing2_K : Outport
  T_MGHousing3_K : Outport  Port=2
  T_MGHousing4_K : Outport  Port=3
  T_MGHousing5_K : Outport  Port=4
  T_MGHousing1_K : Outport  Port=5
  wires:
  PHI_MGHousing1_W/1 -> Add/1
  Constant/1 -> Divide/1
  Add/1 -> Divide/2
  Divide/1 -> Integrator/1
  Temp_ini/1 -> degC->K/1(degC)
  Integrator/1 -> Add1/2
  Add1/1 -> T_MGHousing1_K/1, T_MGHousing2_K/1, T_MGHousing5_K/1, T_MGHousing3_K/1, T_MGHousing4_K/1
  degC->K/1(K) -> Add1/1
  PHI_MGHousing2_W/1 -> Add/2
  PHI_MGHousing3_W/1 -> Add/5
  PHI_MGHousing4_W/1 -> Add/4
  PHI_MGHousing5_W/1 -> Add/3

== system EV_thermal_charger_2015a_20200311/Vehicle/ELTH_PNT/MGTH_PNT/PTTH2MGHousing_Heat_Resistance ==
  T_MGHousing_Resi2_K : Inport
  T_PTTH_Resi2_K : Inport  Port=2
  Add : Sum  Inputs=+-
  Constant : Constant  Value=ELTH_PNT_PTTH2MGHousing_Heat_Resi_KpW
  Divide : Product  Inputs=*/
  Gain : Gain  Gain=-1
  Gain1 : Gain
  PHI_MGHousing_Resi2_W : Outport
  PHI_PTTH_Resi2_W : Outport  Port=2
  wires:
  Constant/1 -> Divide/2
  Add/1 -> Divide/1
  Divide/1 -> Gain1/1, Gain/1
  Gain/1 -> PHI_PTTH_Resi2_W/1
  T_PTTH_Resi2_K/1 -> Add/1
  T_MGHousing_Resi2_K/1 -> Add/2
  Gain1/1 -> PHI_MGHousing_Resi2_W/1

== system EV_thermal_charger_2015a_20200311/Vehicle/ELTH_PNT/RD_PNT/INV2Coolant_Heat_Resistance1 ==
  Qv_Coolant_m3ps : Inport
  T_INVTH_Resi_K : Inport  Port=2
  T_Coolant_Resi_K : Inport  Port=3
  1-D Lookup Table : Lookup_n-D  NumberOfTableDimensions=1  BreakpointsForDimension1=ELTH_PNT_INV2Coolant_Heat_Resi_x_qv_Coolant  Table=ELTH_PNT_INV2Coolant_Heat_Resi_KpW  InternalRulePriority=Speed  RndMeth=Simplest  InputSameDT=on
  Add : Sum  Inputs=+-
  Divide : Product  Inputs=*/
  Gain : Gain  Gain=-1
  Gain1 : Gain
  PHI_Coolant_Resi_W : Outport
  PHI_INVTH_Resi_W : Outport  Port=2
  wires:
  1-D Lookup Table/1 -> Divide/2
  Add/1 -> Divide/1
  Divide/1 -> Gain1/1, Gain/1
  T_Coolant_Resi_K/1 -> Add/2
  T_INVTH_Resi_K/1 -> Add/1
  Gain/1 -> PHI_INVTH_Resi_W/1
  Gain1/1 -> PHI_Coolant_Resi_W/1
  Qv_Coolant_m3ps/1 -> 1-D Lookup Table/1
